simulink model "MultiInv_7lvl"  (R2015a)
settings: Solver=ode45  StartTime=0.0  StopTime=0.08  RelTol=1e-3
values from neighbouring files (symbols this model uses):
  a = a_m(1,1)    [INV_7level.m]    (also in Inv5level.m)
  b = a_m(2,1)    [INV_7level.m]    (also in Inv5level.m)
libraries: powerlib x14
settings Model: Creator=Hp-user  LastModifiedBy=Hp-user

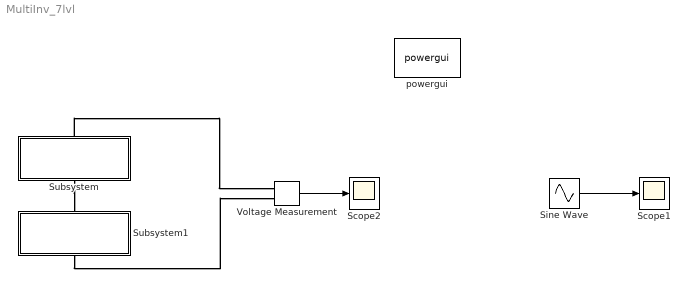
== system MultiInv_7lvl ==
  Scope1 : Scope
      settings: SaveName=sinwave  MaxDataPoints=5000000
  Scope2 : Scope
      settings: SaveName=OutVolt  MaxDataPoints=5000000
  Sine Wave : Sin  Amplitude=60  Frequency=0.2*pi  SampleTime=0
  Subsystem : Subsystem
  Subsystem1 : Subsystem
  Voltage Measurement : powerlib/Measurements/Voltage Measurement  PhasorSimulation=off  OutputType=Complex  PSBequivalent=0
  powergui : powerlib/powergui  Priority=1  SimulationMode=Continuous  SolverType=Tustin/Backward Euler (TBE)  SampleTime=50e-6  frequency=60  SPID=off  DisableSnubberDevices=off  DisableRonSwitches=off  DisableVfSwitches=off  SwTol=0  DisplayEquations=off  Interpol=off  methode=off  Ts=100  FunctionMessages=off  echomessages=off  HookPort=off  EnableUseOfTLC=off  x0status=blocks  frequencyindice=0  Pbase=100e6  ErrMax=1e-4  Iterations=50  UnitsV=kV  UnitsW=MW  buscounter=0  RestoreLinks=warning  ResistiveCurrentMeasurement=off  Frange=[0:2:500]  Ylog=off  Xlog=on  ShowGrid=off  save=off  variable=ZData  structure=OutVolt  ZoomFFT=off  StartTime=0.01  cycles=2  DisplayStyle=2  fundamental=50  FreqAxis=off  MaxFrequency=1000  frequencyindicesteady=1  RmsSteady=1  display=off
  wires:
  Voltage Measurement/1 -> Scope2/1
  Sine Wave/1 -> Scope1/1
  connections:
  Subsystem1/RConn1 -- Voltage Measurement/LConn2
  Subsystem/LConn1 -- Voltage Measurement/LConn1
  Subsystem/RConn1 -- Subsystem1/LConn1

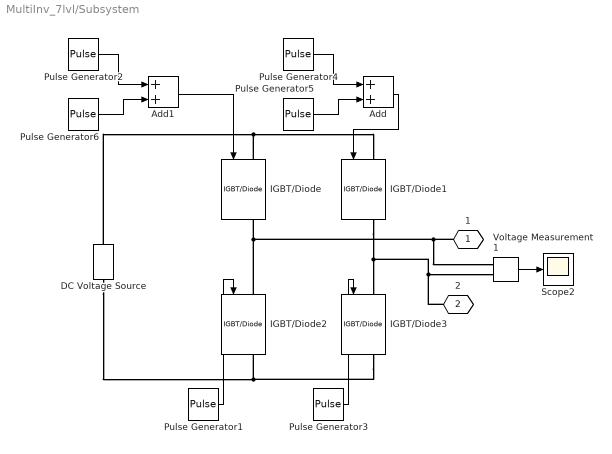
== system MultiInv_7lvl/Subsystem ==
  Add : Sum
  Add1 : Sum
  DC Voltage Source : powerlib/Electrical Sources/DC Voltage Source  Amplitude=12  Measurements=None
  IGBT/Diode{,1..3} (4 alike) : powerlib/Power Electronics/IGBT//Diode  Ron=1e-3  Rs=1e5  Cs=inf  Measurements=on
  Pulse Generator1 : DiscretePulseGenerator  PulseType=Time based  Period=t  PulseWidth=50-((5*a)/9)  PhaseDelay=((180+a)*t)/360
  Pulse Generator2 : DiscretePulseGenerator  PulseType=Time based  Period=t  PulseWidth=50+((5*a)/18)
  Pulse Generator3 : DiscretePulseGenerator  PulseType=Time based  Period=t  PulseWidth=50-((5*a)/9)  PhaseDelay=(a*t)/360
  Pulse Generator4 : DiscretePulseGenerator  PulseType=Time based  Period=t  PulseWidth=a/3.6
  Pulse Generator5 : DiscretePulseGenerator  PulseType=Time based  Period=t  PulseWidth=50+((5*a)/18)  PhaseDelay=(180-a)*(t/360)
  Pulse Generator6 : DiscretePulseGenerator  PulseType=Time based  Period=t  PulseWidth=a/3.6  PhaseDelay=(360-a)*(t/360)
  Scope2 : Scope
      settings: SaveName=ScopeData6
  Voltage Measurement1 : powerlib/Measurements/Voltage Measurement  PhasorSimulation=off  OutputType=Complex  PSBequivalent=0
  1 : PMIOPort  Tag=PMCPort  Port=1  Side=Left
  2 : PMIOPort  Tag=PMCPort  Port=2  Side=Right
  wires:
  Pulse Generator1/1 -> IGBT/Diode2/1
  Pulse Generator3/1 -> IGBT/Diode3/1
  Pulse Generator4/1 -> Add/1
  Pulse Generator5/1 -> Add/2
  Add/1 -> IGBT/Diode1/1
  Voltage Measurement1/1 -> Scope2/1
  Pulse Generator2/1 -> Add1/1
  Pulse Generator6/1 -> Add1/2
  Add1/1 -> IGBT/Diode/1
  connections:
  DC Voltage Source/LConn1 -- IGBT/Diode3/RConn1 -- IGBT/Diode2/RConn1
  DC Voltage Source/RConn1 -- IGBT/Diode/LConn1 -- IGBT/Diode1/LConn1
  2/RConn1 -- IGBT/Diode1/RConn1 -- IGBT/Diode3/LConn1 -- Voltage Measurement1/LConn2
  1/RConn1 -- IGBT/Diode2/LConn1 -- IGBT/Diode/RConn1 -- Voltage Measurement1/LConn1

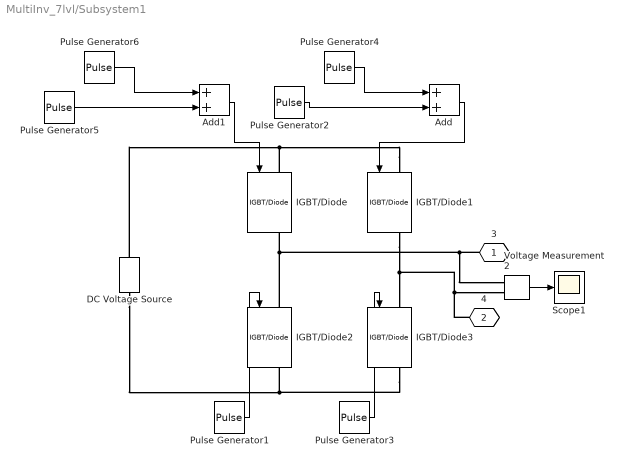
== system MultiInv_7lvl/Subsystem1 ==
  Add : Sum
  Add1 : Sum
  DC Voltage Source : powerlib/Electrical Sources/DC Voltage Source  Amplitude=12  Measurements=None
  IGBT/Diode{,1..3} (4 alike) : powerlib/Power Electronics/IGBT//Diode  Ron=1e-3  Rs=1e5  Cs=inf  Measurements=on
  Pulse Generator1 : DiscretePulseGenerator  PulseType=Time based  Period=t  PulseWidth=50-((5*b)/9)  PhaseDelay=((180+b)*t)/360
  Pulse Generator2 : DiscretePulseGenerator  PulseType=Time based  Period=t  PulseWidth=50+((5*b)/18)  PhaseDelay=(180-b)*(t/360)
  Pulse Generator3 : DiscretePulseGenerator  PulseType=Time based  Period=t  PulseWidth=50-((5*b)/9)  PhaseDelay=(b*t)/360
  Pulse Generator4 : DiscretePulseGenerator  PulseType=Time based  Period=t  PulseWidth=b/3.6
  Pulse Generator5 : DiscretePulseGenerator  PulseType=Time based  Period=t  PulseWidth=b/3.6  PhaseDelay=(360-b)*(t/360)
  Pulse Generator6 : DiscretePulseGenerator  PulseType=Time based  Period=t  PulseWidth=50+((5*b)/18)
  Scope1 : Scope
      settings: SaveName=ScopeData5
  Voltage Measurement2 : powerlib/Measurements/Voltage Measurement  PhasorSimulation=off  OutputType=Complex  PSBequivalent=0
  3 : PMIOPort  Tag=PMCPort  Port=1  Side=Left
  4 : PMIOPort  Tag=PMCPort  Port=2  Side=Right
  wires:
  Add/1 -> IGBT/Diode1/1
  Pulse Generator2/1 -> Add/2
  Pulse Generator4/1 -> Add/1
  Pulse Generator3/1 -> IGBT/Diode3/1
  Pulse Generator1/1 -> IGBT/Diode2/1
  Voltage Measurement2/1 -> Scope1/1
  Add1/1 -> IGBT/Diode/1
  Pulse Generator5/1 -> Add1/2
  Pulse Generator6/1 -> Add1/1
  connections:
  3/RConn1 -- IGBT/Diode/RConn1 -- IGBT/Diode2/LConn1 -- Voltage Measurement2/LConn1
  4/RConn1 -- IGBT/Diode3/LConn1 -- IGBT/Diode1/RConn1 -- Voltage Measurement2/LConn2
  IGBT/Diode1/LConn1 -- DC Voltage Source/RConn1 -- IGBT/Diode/LConn1
  IGBT/Diode2/RConn1 -- IGBT/Diode3/RConn1 -- DC Voltage Source/LConn1
